simulink model "gm_sampleModel1965_4_sub"  (R2023a)
settings: Solver=VariableStepAuto  StartTime=0.0  StopTime=10.0  RelTol=1e-3
libraries: simulink x1, hdlsllib x1
settings Model: Creator=user1  LastModifiedBy=user1
settings OptimizationCC: BlockReduction=off  ConditionallyExecuteInputs=off
settings DebuggingCC: InheritedTsInSrcMsg=none

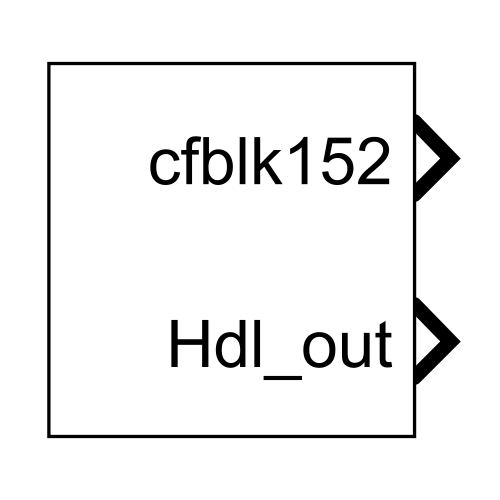
[thumbnail: Simulink's stored preview of the top-level diagram]
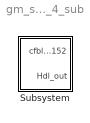
== system gm_sampleModel1965_4_sub ==
  Subsystem : Subsystem

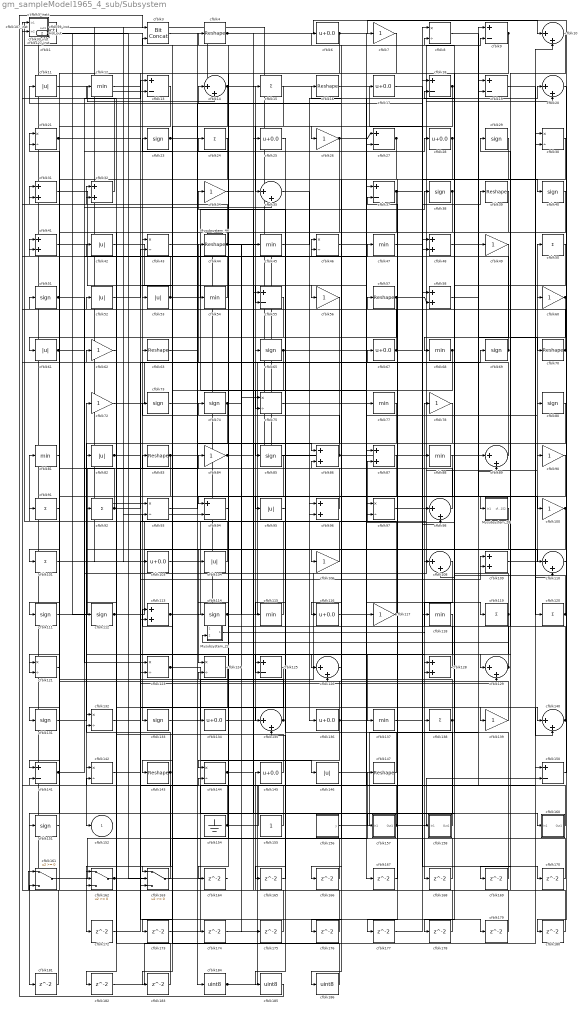
== system gm_sampleModel1965_4_sub/Subsystem ==
  Mysubsystem_22 : Subsystem
  Mysubsystem_28 : Subsystem
  Mysubsystem_44 : Subsystem
  cfblk1 : simulink/Logic and Bit Operations/Extract Bits  bitsToExtract=Upper half  numBits=8  bitIdxRange=[0 7]  outScalingMode=Preserve fixed-point scaling
      settings: LibrarySourceBlock=|
      | hdlsllib/Logic and Bit
      | Operations/Extract Bits
  cfblk{10,14,20,35,89,98,108,110,126,129,135,140} (12 alike) : Sum  Inputs=|++  OutDataTypeStr=uint8
  cfblk{7,26,34,49,56,60,62,72,78,84,90,100,106,117,139} (15 alike) : Gain  OutDataTypeStr=uint8
  cfblk{15,24,50,91..92,101,119..120,138} (9 alike) : Sum  Inputs=+  OutDataTypeStr=uint8
  cfblk102_inst : Subsystem
  cfblk{6,17,25,28,67,103,116,134,136,145} (10 alike) : Bias  Bias=0.0  SaturateOnIntegerOverflow=off
  cfblk{11,42,52..53,61,82,95,104,146} (9 alike) : Abs  OutDataTypeStr=uint8  SaturateOnIntegerOverflow=off
  cfblk107_inst : Subsystem
  cfblk{31..32,41,48,58,86..87,96,109,113,128} (11 alike) : Sum  OutDataTypeStr=uint8
  cfblk{23,29,38,40,51,65,69,73..74,80,85,111..112,114,131,133,151} (17 alike) : Signum
  cfblk{12,45,47,54,68,77,81,88,115,118,137} (11 alike) : MinMax  OutDataTypeStr=uint8
  cfblk{8,21,30,43,46,75,93,97,121,123..124,132,142,144} (14 alike) : Product  Inputs=*/  OutDataTypeStr=uint8  RndMeth=Zero  SaturateOnIntegerOverflow=on
  cfblk{9,13,18..19,27,37,55,94,125,141,150} (11 alike) : Sum  Inputs=+-  OutDataTypeStr=uint8
  cfblk127_inst : Subsystem
  cfblk{4,16,39,44,57,63,70,83,143,147} (10 alike) : Reshape
  cfblk154 : Ground
  cfblk155 : Constant  OutDataTypeStr=uint8  SampleTime=-1
  cfblk156 : Subsystem  mask(Counter Limited){uplimit=double(7), tsamp=double(-1)}
      mask prompts: uplimit "Simulink:masks:UpperLimit_MP"; tsamp "Simulink:masks:SampleTime_MP"
      mask help: Simulink:masks:CounterLimited_MD
      mask init:
      | nbits = double(8);
      | tsamp = double(-1);
      | uplimit = double(7);
  cfblk157 : Subsystem
  cfblk158 : Subsystem
  cfblk160 : Subsystem
  cfblk161 : Switch  OutDataTypeStr=uint8  SaturateOnIntegerOverflow=off  InputSameDT=off
  cfblk162 : Switch  OutDataTypeStr=uint8  SaturateOnIntegerOverflow=off  InputSameDT=off
  cfblk163 : Switch  OutDataTypeStr=uint8  SaturateOnIntegerOverflow=off  InputSameDT=off
  cfblk{164..170,172..183} (19 alike) : Delay  SampleTime=1
  cfblk184 : DataTypeConversion  OutDataTypeStr=uint8  SaturateOnIntegerOverflow=off  RndMeth=Floor
  cfblk185 : DataTypeConversion  OutDataTypeStr=uint8  SaturateOnIntegerOverflow=off  RndMeth=Floor
  cfblk186 : DataTypeConversion  OutDataTypeStr=uint8  SaturateOnIntegerOverflow=off  RndMeth=Floor
  cfblk3 : hdlsllib/Logic and Bit Operations/Bit Concat  numInputs=2
  cfblk33_inst : Subsystem
  cfblk59_inst : Subsystem
  cfblk5_inst : Subsystem
  cfblk152 : Outport  OutDataTypeStr=uint8  SampleTime=1  VectorParamsAs1DForOutWhenUnconnected=off
  Hdl_out : Outport  Port=2  OutDataTypeStr=uint8  SampleTime=1
  wires:
  Mysubsystem_22/1(Out1) -> cfblk168/1
  Mysubsystem_28/1(cfblk152) -> cfblk152/1
  Mysubsystem_44/1(Out1) -> Mysubsystem_22/1(In1)
  cfblk1/1 -> cfblk133/1
  cfblk10/1 -> cfblk145/1
  cfblk100/1 -> cfblk108/2, cfblk124/1
  cfblk101/1 -> cfblk106/1
  cfblk102_inst/1(out1) -> cfblk13/2, cfblk93/1
  cfblk103/1 -> cfblk143/1
  cfblk104/1 -> cfblk81/1
  cfblk106/1 -> cfblk15/1
  cfblk107_inst/1(out1) -> cfblk94/2
  cfblk108/1 -> cfblk138/1
  cfblk109/1 -> cfblk50/1
  cfblk11/1 -> cfblk14/2
  cfblk110/1 -> cfblk7/1
  cfblk111/1 -> cfblk83/1
  cfblk112/1 -> cfblk90/1, Hdl_out/1
  cfblk113/1 -> cfblk9/2, cfblk20/2
  cfblk114/1 -> cfblk67/1, cfblk45/1
  cfblk115/1 -> cfblk102_inst/1(in1)
  cfblk116/1 -> cfblk117/1
  cfblk117/1 -> cfblk87/2, cfblk23/1
  cfblk118/1 -> cfblk142/1
  cfblk119/1 -> cfblk97/2, cfblk137/1
  cfblk12/1 -> cfblk55/2
  cfblk120/1 -> cfblk127_inst/2(in2), cfblk109/1, cfblk8/2
  cfblk121/1 -> cfblk41/1
  cfblk123/1 -> cfblk146/1, cfblk160/1(In1)
  cfblk124/1 -> cfblk163/1
  cfblk125/1 -> cfblk182/1
  cfblk126/1 -> cfblk176/1
  cfblk127_inst/1(out1) -> cfblk103/1
  cfblk128/1 -> cfblk78/1
  cfblk129/1 -> Mysubsystem_22/2(In2), cfblk24/1
  cfblk13/1 -> cfblk101/1
  cfblk131/1 -> cfblk72/1
  cfblk132/1 -> cfblk97/1
  cfblk133/1 -> cfblk30/1
  cfblk134/1 -> cfblk65/1
  cfblk135/1 -> cfblk4/1, cfblk31/1
  cfblk136/1 -> cfblk20/1, cfblk21/1, cfblk144/1
  cfblk137/1 -> cfblk88/1
  cfblk138/1 -> cfblk11/1, cfblk181/1
  cfblk139/1 -> cfblk41/2
  cfblk14/1 -> cfblk129/2, cfblk173/1
  cfblk140/1 -> cfblk74/1, cfblk29/1
  cfblk141/1 -> cfblk35/2, cfblk108/1, cfblk84/1, cfblk47/1
  cfblk142/1 -> cfblk126/2
  cfblk143/1 -> cfblk172/1, cfblk132/2
  cfblk144/1 -> cfblk38/1, cfblk46/1
  cfblk145/1 -> cfblk12/1
  cfblk146/1 -> cfblk19/2
  cfblk147/1 -> cfblk34/1
  cfblk15/1 -> cfblk35/1
  cfblk150/1 -> cfblk60/1
  cfblk151/1 -> cfblk91/1
  cfblk154/1 -> cfblk5_inst/1(in1), cfblk27/2
  cfblk155/1 -> cfblk113/1
  cfblk156/1(y) -> cfblk58/1
  cfblk157/1(Out1) -> cfblk16/1, cfblk150/2
  cfblk158/1(Out1) -> cfblk52/1
  cfblk16/1 -> cfblk118/1
  cfblk160/1(Out1) -> cfblk142/2
  cfblk161/1 -> cfblk147/1
  cfblk162/1 -> cfblk109/2, cfblk62/1
  cfblk163/1 -> cfblk33_inst/1(in1)
  cfblk164/1 -> cfblk1/1
  cfblk165/1 -> cfblk135/2
  cfblk166/1 -> cfblk93/2
  cfblk167/1 -> cfblk37/2
  cfblk168/1 -> cfblk86/2
  cfblk169/1 -> cfblk18/2
  cfblk17/1 -> cfblk98/2
  cfblk170/1 -> cfblk124/2
  cfblk172/1 -> cfblk144/2
  cfblk173/1 -> cfblk8/1
  cfblk174/1 -> cfblk10/2
  cfblk175/1 -> cfblk102_inst/2(in2)
  cfblk176/1 -> cfblk161/3
  cfblk177/1 -> cfblk48/2
  cfblk178/1 -> cfblk33_inst/2(in2)
  cfblk179/1 -> cfblk141/2
  cfblk18/1 -> cfblk26/1, cfblk164/1
  cfblk180/1 -> cfblk55/1
  cfblk181/1 -> cfblk161/1
  cfblk182/1 -> cfblk30/2
  cfblk183/1 -> cfblk32/1
  cfblk184/1 -> cfblk89/2, cfblk150/1, cfblk49/1
  cfblk185/1 -> cfblk3/1
  cfblk186/1 -> cfblk3/2
  cfblk19/1 -> cfblk120/1
  cfblk20/1 -> cfblk180/1
  cfblk21/1 -> cfblk113/2, cfblk179/1
  cfblk23/1 -> cfblk134/1, Mysubsystem_28/1(In1)
  cfblk24/1 -> cfblk43/1
  cfblk25/1 -> cfblk125/2
  cfblk26/1 -> cfblk27/1, cfblk140/1, cfblk121/2
  cfblk27/1 -> cfblk111/1, cfblk75/2
  cfblk28/1 -> cfblk126/1, cfblk177/1
  cfblk29/1 -> cfblk63/1
  cfblk3/1 -> cfblk184/1
  cfblk30/1 -> cfblk53/1
  cfblk31/1 -> cfblk77/1
  cfblk32/1 -> cfblk5_inst/2(in2)
  cfblk33_inst/1(out1) -> cfblk104/1
  cfblk34/1 -> cfblk86/1
  cfblk35/1 -> cfblk96/1
  cfblk37/1 -> cfblk48/1, cfblk40/1, cfblk163/3
  cfblk38/1 -> cfblk186/1, cfblk162/3
  cfblk39/1 -> cfblk115/1
  cfblk4/1 -> cfblk25/1, cfblk10/1
  cfblk40/1 -> cfblk125/1
  cfblk41/1 -> cfblk136/1
  cfblk42/1 -> cfblk56/1
  cfblk43/1 -> cfblk167/1
  cfblk44/1 -> cfblk59_inst/2(in2), cfblk175/1
  cfblk45/1 -> cfblk19/1
  cfblk46/1 -> cfblk87/1
  cfblk47/1 -> cfblk39/1
  cfblk48/1 -> cfblk70/1
  cfblk49/1 -> cfblk68/1
  cfblk5_inst/1(out1) -> cfblk161/2
  cfblk50/1 -> cfblk158/1(In1)
  cfblk51/1 -> cfblk46/2, cfblk123/1
  cfblk52/1 -> cfblk43/2
  cfblk53/1 -> cfblk37/1, cfblk31/2
  cfblk54/1 -> cfblk59_inst/1(in1)
  cfblk55/1 -> cfblk123/2
  cfblk56/1 -> cfblk132/1
  cfblk57/1 -> cfblk58/2, cfblk131/1
  cfblk58/1 -> cfblk9/1
  cfblk59_inst/1(out1) -> cfblk89/1, cfblk17/1
  cfblk6/1 -> cfblk163/2, cfblk119/1
  cfblk60/1 -> cfblk129/1, cfblk169/1
  cfblk61/1 -> cfblk28/1, cfblk13/1
  cfblk62/1 -> cfblk82/1
  cfblk63/1 -> cfblk174/1
  cfblk65/1 -> cfblk183/1, cfblk139/1
  cfblk67/1 -> cfblk98/1, cfblk107_inst/2(in2)
  cfblk68/1 -> cfblk95/1, cfblk166/1
  cfblk69/1 -> cfblk57/1, cfblk107_inst/1(in1)
  cfblk7/1 -> cfblk94/1
  cfblk70/1 -> cfblk6/1, cfblk32/2
  cfblk72/1 -> cfblk44/1
  cfblk73/1 -> cfblk135/1
  cfblk74/1 -> cfblk112/1, cfblk75/1
  cfblk75/1 -> cfblk110/1
  cfblk77/1 -> cfblk116/1
  cfblk78/1 -> cfblk96/2
  cfblk8/1 -> cfblk100/1
  cfblk80/1 -> cfblk114/1
  cfblk81/1 -> cfblk141/1
  cfblk82/1 -> cfblk140/2, cfblk128/2, cfblk128/1
  cfblk83/1 -> cfblk85/1, cfblk162/2
  cfblk84/1 -> cfblk110/2, cfblk157/1(In1)
  cfblk85/1 -> cfblk121/1
  cfblk86/1 -> cfblk80/1, cfblk73/1, Mysubsystem_44/1(In1)
  cfblk87/1 -> cfblk92/1
  cfblk88/1 -> cfblk151/1
  cfblk89/1 -> cfblk127_inst/1(in1)
  cfblk9/1 -> cfblk61/1, cfblk178/1
  cfblk90/1 -> cfblk185/1
  cfblk91/1 -> cfblk51/1
  cfblk92/1 -> cfblk69/1, cfblk162/1, cfblk21/2
  cfblk93/1 -> cfblk18/1
  cfblk94/1 -> cfblk14/1
  cfblk95/1 -> cfblk165/1
  cfblk96/1 -> cfblk54/1
  cfblk97/1 -> cfblk170/1
  cfblk98/1 -> cfblk42/1

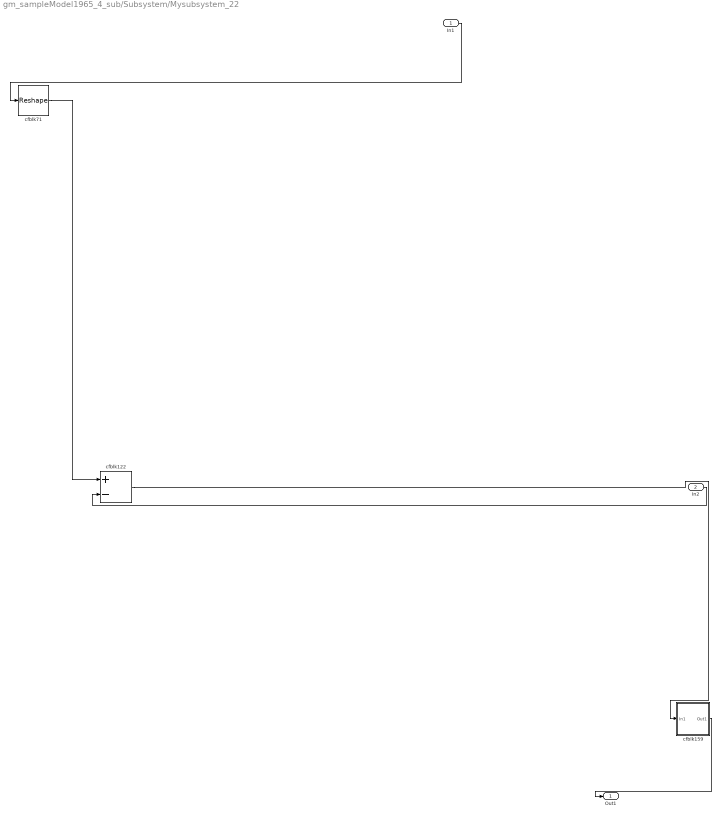
== system gm_sampleModel1965_4_sub/Subsystem/Mysubsystem_22 ==
  In1 : Inport  OutDataTypeStr=uint8  PortDimensions=1  SampleTime=1
  In2 : Inport  Port=2  OutDataTypeStr=uint8  PortDimensions=1  SampleTime=1
  cfblk122 : Sum  Inputs=+-
  cfblk159 : Subsystem
  cfblk71 : Reshape
  Out1 : Outport  SampleTime=1
  wires:
  In1/1 -> cfblk71/1
  In2/1 -> cfblk122/2
  cfblk122/1 -> cfblk159/1(In1)
  cfblk159/1(Out1) -> Out1/1
  cfblk71/1 -> cfblk122/1

== system gm_sampleModel1965_4_sub/Subsystem/Mysubsystem_28 ==
  In1 : Inport  OutDataTypeStr=uint8  PortDimensions=1  SampleTime=1
  cfblk99 : Sum  Inputs=+
  cfblk152 : Outport  SampleTime=1  VectorParamsAs1DForOutWhenUnconnected=off
  wires:
  In1/1 -> cfblk99/1
  cfblk99/1 -> cfblk152/1

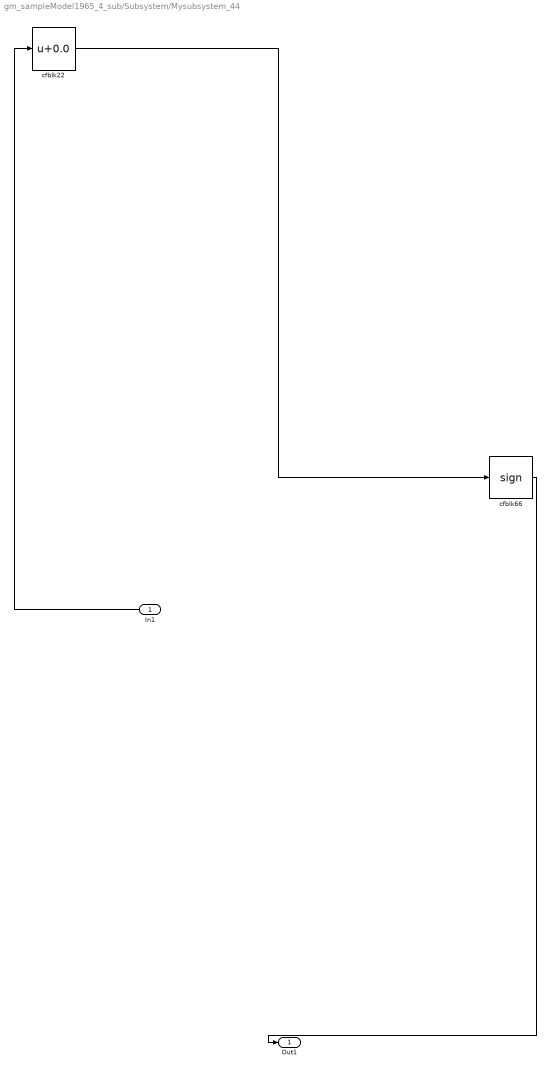
== system gm_sampleModel1965_4_sub/Subsystem/Mysubsystem_44 ==
  In1 : Inport  OutDataTypeStr=uint8  PortDimensions=1  SampleTime=1
  cfblk22 : Bias  Bias=0.0  SaturateOnIntegerOverflow=off
  cfblk66 : Signum
  Out1 : Outport  SampleTime=1
  wires:
  In1/1 -> cfblk22/1
  cfblk22/1 -> cfblk66/1
  cfblk66/1 -> Out1/1

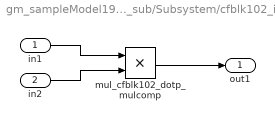
== system gm_sampleModel1965_4_sub/Subsystem/cfblk102_inst ==
  in1 : Inport  OutDataTypeStr=uint8  SampleTime=1
  in2 : Inport  Port=2  OutDataTypeStr=uint8  SampleTime=1
  mul_cfblk102_dotp_mulcomp : Product  Inputs=**  OutDataTypeStr=uint8  SampleTime=1
  out1 : Outport  OutDataTypeStr=uint8  SampleTime=1
  wires:
  in1/1 -> mul_cfblk102_dotp_mulcomp/1
  in2/1 -> mul_cfblk102_dotp_mulcomp/2
  mul_cfblk102_dotp_mulcomp/1 -> out1/1

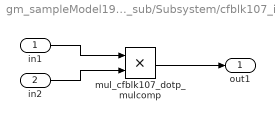
== system gm_sampleModel1965_4_sub/Subsystem/cfblk107_inst ==
  in1 : Inport  OutDataTypeStr=uint8  SampleTime=1
  in2 : Inport  Port=2  OutDataTypeStr=uint8  SampleTime=1
  mul_cfblk107_dotp_mulcomp : Product  Inputs=**  OutDataTypeStr=uint8  SampleTime=1
  out1 : Outport  OutDataTypeStr=uint8  SampleTime=1
  wires:
  in1/1 -> mul_cfblk107_dotp_mulcomp/1
  in2/1 -> mul_cfblk107_dotp_mulcomp/2
  mul_cfblk107_dotp_mulcomp/1 -> out1/1

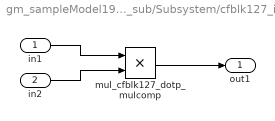
== system gm_sampleModel1965_4_sub/Subsystem/cfblk127_inst ==
  in1 : Inport  OutDataTypeStr=uint8  SampleTime=1
  in2 : Inport  Port=2  OutDataTypeStr=uint8  SampleTime=1
  mul_cfblk127_dotp_mulcomp : Product  Inputs=**  OutDataTypeStr=uint8  SampleTime=1
  out1 : Outport  OutDataTypeStr=uint8  SampleTime=1
  wires:
  in1/1 -> mul_cfblk127_dotp_mulcomp/1
  in2/1 -> mul_cfblk127_dotp_mulcomp/2
  mul_cfblk127_dotp_mulcomp/1 -> out1/1

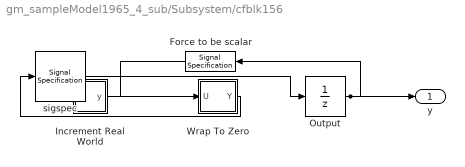
== system gm_sampleModel1965_4_sub/Subsystem/cfblk156 ==
  Force to be scalar : SignalSpecification  DisableCoverage=on  Dimensions=1
  Increment Real World : Subsystem  mask(Real World Value Increment){}
      mask help: Simulink:masks:RealWorldValueIncrement_MD
      mask Display: disp('V++')
  Output : UnitDelay  InitialCondition=0.0  SampleTime=tsamp  HasFrameUpgradeWarning=on
  Wrap To Zero : Subsystem  mask(Wrap To Zero){Threshold=double(7)}
      mask prompts: Threshold "Simulink:masks:Threshold_MP"
      mask help: Simulink:masks:WrapToZero_MD
  sigspec : SignalSpecification  OutDataTypeStr=uint8  Dimensions=1
  y : Outport  SampleTime=1
  wires:
  Force to be scalar/1 -> Increment Real World/1(u)
  Increment Real World/1(y) -> Wrap To Zero/1(U)
  Output/1 -> Force to be scalar/1, y/1
  Wrap To Zero/1(Y) -> sigspec/1
  sigspec/1 -> Output/1

== system gm_sampleModel1965_4_sub/Subsystem/cfblk157 ==
  In1 : Inport  OutDataTypeStr=uint8  PortDimensions=1  SampleTime=1
  Out1 : Outport  SampleTime=1
  wires:
  In1/1 -> Out1/1

== system gm_sampleModel1965_4_sub/Subsystem/cfblk158 ==
  In1 : Inport  OutDataTypeStr=uint8  PortDimensions=1  SampleTime=1
  Out1 : Outport  SampleTime=1
  wires:
  In1/1 -> Out1/1

== system gm_sampleModel1965_4_sub/Subsystem/cfblk160 ==
  In1 : Inport  OutDataTypeStr=uint8  PortDimensions=1  SampleTime=1
  Out1 : Outport  SampleTime=1
  wires:
  In1/1 -> Out1/1

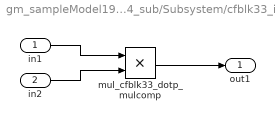
== system gm_sampleModel1965_4_sub/Subsystem/cfblk33_inst ==
  in1 : Inport  OutDataTypeStr=uint8  SampleTime=1
  in2 : Inport  Port=2  OutDataTypeStr=uint8  SampleTime=1
  mul_cfblk33_dotp_mulcomp : Product  Inputs=**  OutDataTypeStr=uint8  SampleTime=1
  out1 : Outport  OutDataTypeStr=uint8  SampleTime=1
  wires:
  in1/1 -> mul_cfblk33_dotp_mulcomp/1
  in2/1 -> mul_cfblk33_dotp_mulcomp/2
  mul_cfblk33_dotp_mulcomp/1 -> out1/1

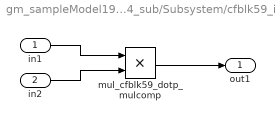
== system gm_sampleModel1965_4_sub/Subsystem/cfblk59_inst ==
  in1 : Inport  OutDataTypeStr=uint8  SampleTime=1
  in2 : Inport  Port=2  OutDataTypeStr=uint8  SampleTime=1
  mul_cfblk59_dotp_mulcomp : Product  Inputs=**  OutDataTypeStr=uint8  SampleTime=1
  out1 : Outport  OutDataTypeStr=uint8  SampleTime=1
  wires:
  in1/1 -> mul_cfblk59_dotp_mulcomp/1
  in2/1 -> mul_cfblk59_dotp_mulcomp/2
  mul_cfblk59_dotp_mulcomp/1 -> out1/1

== system gm_sampleModel1965_4_sub/Subsystem/cfblk5_inst ==
  in1 : Inport  OutDataTypeStr=uint8  SampleTime=1
  in2 : Inport  Port=2  OutDataTypeStr=uint8  SampleTime=1
  mul_cfblk5_dotp_mulcomp : Product  Inputs=**  OutDataTypeStr=uint8  SampleTime=1
  out1 : Outport  OutDataTypeStr=uint8  SampleTime=1
  wires:
  in1/1 -> mul_cfblk5_dotp_mulcomp/1
  in2/1 -> mul_cfblk5_dotp_mulcomp/2
  mul_cfblk5_dotp_mulcomp/1 -> out1/1

== system gm_sampleModel1965_4_sub/Subsystem/Mysubsystem_22/cfblk159 ==
  In1 : Inport  OutDataTypeStr=uint8  PortDimensions=1  SampleTime=1
  Out1 : Outport  SampleTime=1
  wires:
  In1/1 -> Out1/1

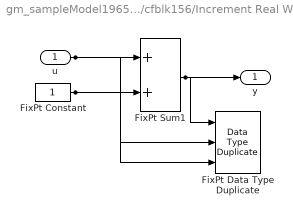
== system gm_sampleModel1965_4_sub/Subsystem/cfblk156/Increment Real World ==
  u : Inport  OutDataTypeStr=uint8  SampleTime=1
  FixPt Constant : Constant  DisableCoverage=on  OutDataTypeStr=Inherit: Inherit via back propagation  SampleTime=-1
  FixPt Data Type Duplicate : DataTypeDuplicate  DisableCoverage=on  NumInputPorts=3
  FixPt Sum1 : Sum  InputSameDT=on  OutDataTypeStr=Inherit: Inherit via back propagation  LockScale=on
  y : Outport  SampleTime=1
  wires:
  u/1 -> FixPt Sum1/1, FixPt Data Type Duplicate/2
  FixPt Constant/1 -> FixPt Sum1/2, FixPt Data Type Duplicate/3
  FixPt Sum1/1 -> FixPt Data Type Duplicate/1, y/1

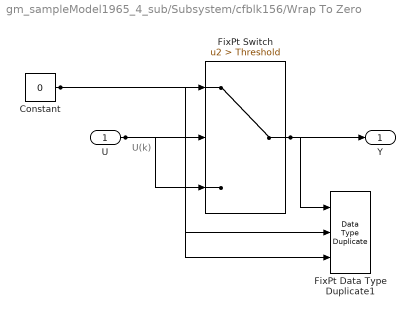
== system gm_sampleModel1965_4_sub/Subsystem/cfblk156/Wrap To Zero ==
  note: U(k)
  U : Inport  OutDataTypeStr=uint8  SampleTime=1
  Constant : Constant  DisableCoverage=on  Value=0  OutDataTypeStr=Inherit: Inherit via back propagation  SampleTime=-1
  FixPt Data Type Duplicate1 : DataTypeDuplicate  DisableCoverage=on  NumInputPorts=3
  FixPt Switch : Switch  Criteria=u2 > Threshold  Threshold=Threshold  OutDataTypeStr=Inherit: Inherit via back propagation  ZeroCross=off  SaturateOnIntegerOverflow=off  InputSameDT=off
  Y : Outport  SampleTime=1
  wires:
  U/1 -> FixPt Switch/3, FixPt Switch/2, FixPt Data Type Duplicate1/2
  Constant/1 -> FixPt Switch/1, FixPt Data Type Duplicate1/3
  FixPt Switch/1 -> FixPt Data Type Duplicate1/1, Y/1
